simulink model "Sim_Multi"  (R2016b)
settings: Solver=ode3  StartTime=0.0  StopTime=sim_time  FixedStep=t_sim  MaxStep=t_control  RelTol=1e-5  EnableMultiTasking=on
values from neighbouring files (symbols this model uses):
  Att_init = [0;0;0] * d2r    [Init_Multi.m]
  Blade_flapping = 0    [Init_Multi.m]
  C_D = 0.40    (= 0.4)    [Init_Multi.m]
  CoG_nominal = [0;0;0.001]    [Init_Multi.m]
  CoG_real = [0;0;0.001]    [Init_Multi.m]
  Coriolis_correction = 1    [Init_Multi.m]
  d2r = pi/180    (= 0.0174532925199)    [Init_Multi.m]
  Dyn_thrust = 0    [Init_Multi.m]
  g = 9.80665    [Init_Multi.m]
  J_nominal = [Jxx Jxy Jxz;Jyx Jyy Jyz;Jzx Jzy Jzz]    [Init_Multi.m]
  J_real = [Jxx Jxy Jxz;Jyx Jyy Jyz;Jzx Jzy Jzz]    [Init_Multi.m]
  k1 = -1.125    [Init_Multi.m]
  k2 = -1.372    [Init_Multi.m]
  k3 = -1.718    [Init_Multi.m]
  k4 = -0.655    [Init_Multi.m]
  k_a1s = 1.5 / 4.0    (= 0.375)    [Init_Multi.m]
  k_beta = 0.23    [Init_Multi.m]
  kappa = 1.00    (= 1)    [Init_Multi.m]
  Kff_1 = 0.7*[1;1;0.95]    [Init_Multi.m]
  Ki_1 = 10*[1;1;1.5]    [Init_Multi.m]
  Kp_1 = 15*[1;1;1.5]    [Init_Multi.m]
  mass_nominal = 0.550    (= 0.55)    [Init_Multi.m]
  mass_real = 0.550    (= 0.55)    [Init_Multi.m]
  max_thrust = max_thrust + (MotorMatrix_nominal(i,7)*MotorMatrix_nominal(i,12)+MotorMatrix_nominal(i,8)*MotorMatrix_nominal(i,12)^2)    [Init_Multi.m]
  MaxRate_cmd = [360;360;120] * d2r    [Init_Multi.m]
  min_thrust = min_thrust + (MotorMatrix_nominal(i,7)*MotorMatrix_nominal(i,11)+MotorMatrix_nominal(i,8)*MotorMatrix_nominal(i,11)^2)    [Init_Multi.m]
  MotorMap = B' * inv(B * B')    [Init_Multi.m]
  MotorMatrix_nominal = [045 , 0.170 , -0.028 , -1 , 1.0 , 0.010 , [9.6820 , 0.010872]*1e-5 , [1.4504 , 0.0016312]*1e-6 , 0000 , 6000 , [0.0 , 0.0 , 0.0] , 8*2.54/100 , 11/1000;                         135 , 0.170 , -0.028 , +1 , 1.0 , 0.010 , [9.6820 , 0.010872]*1e-5 , [1.4504 , 0.0016312]*1e-6 , 0000 , 6000 , [0.0 , 0.0 , 0.0] , 8*2.54/100 , 11/1000;                         225 , 0.170 , -0.028 , -1 , 1.0 , 0.010 , [9. ...(+284 chars)    [Init_Multi.m]
  MotorMatrix_real = [045 , 0.170 , -0.028 , -1 , 1.0 , 0.010 , [9.6820 , 0.010872]*1e-5 , [1.4504 , 0.0016312]*1e-6 , 0000 , 6000 , [0.0 , 0.0 , 0.0] , 8*2.54/100 , 11/1000;                      135 , 0.170 , -0.028 , +1 , 1.0 , 0.010 , [9.6820 , 0.010872]*1e-5 , [1.4504 , 0.0016312]*1e-6 , 0000 , 6000 , [0.0 , 0.0 , 0.0] , 8*2.54/100 , 11/1000;                      225 , 0.170 , -0.028 , -1 , 1.0 , 0.010 , [9.6820 , ...(+275 chars)    [Init_Multi.m]
  Noise_flag = 0    [Init_Multi.m]
  omega_init = [0;0;0]    [Init_Multi.m]
  q_init = rpy2quat(Att_init)    [Init_Multi.m]
  r2d = 180/pi    (= 57.2957795131)    [Init_Multi.m]
  rho = 1.225    [Init_Multi.m]
  rpm2radpersec = 2*pi/60    (= 0.10471975512)    [Init_Multi.m]
  rpm_init = 3104.5025852    [Init_Multi.m]
  Surface_params = [a;b;c]    [Init_Multi.m]
  t_control = 1/500    (= 0.002)    [Init_Multi.m]
  t_sim = t_control/2    (= 0.001)    [Init_Multi.m]
  thrust_gain = (max_thrust - min_thrust) / 1000    (= 0)    [Init_Multi.m]
  thrust_offset = min_thrust    (= 0)    [Init_Multi.m]
  thrust_reserve = 0.10    (= 0.1)    [Init_Multi.m]
  v_h = 4.0    (= 4)    [Init_Multi.m]
  Vb_init = [0;0;0]    [Init_Multi.m]
  Vi_init = R_IB_init' * Vb_init    [Init_Multi.m]
  Xi_init = [0;0;0]    [Init_Multi.m]
undefined symbols (not defined in the file or in its folder): DiscIntNeverNeededParam, rpy2quat, thrust2rpm
libraries: simulink x17
(part 2 of 4)

== system Sim_Multi/True dynamic system representation of a multirotor UAV/Force//Moment computation/Forces and moments generated by spinning propellers ==
  note: Computation of forces and moments for each actuator specified in the initialization routine
  RPM_commands : Inport
  Dynamic parameters : Inport  Port=2
  6DOF dynamics : Inport  Port=3
  Bus Selector : BusSelector  OutputSignals=omega,V_b,DCM_ib
  Bus Selector1 : BusSelector  OutputSignals=Wind_i,MotorMatrix_real,CoG_real
  For Each Subsystem : Subsystem  TreatAsAtomicUnit=on
  Reshape : Reshape  OutputDimensionality=Column vector (2-D)
  Sum of Elements : Sum  Inputs=+  CollapseMode=Specified dimension  CollapseDim=2
  Sum of Elements1 : Sum  Inputs=+  CollapseMode=Specified dimension  CollapseDim=2
  Total airspeed (Body axes) : Subsystem
  Motor moments : Outport
  Motor forces : Outport  Port=2
  tag scope: RPM_motor=global
  wires:
  For Each Subsystem/1(Motor_force) -> Sum of Elements/1
  For Each Subsystem/2(Motor_moment) -> Sum of Elements1/1
  Sum of Elements/1 -> Motor forces/1
  Sum of Elements1/1 -> Motor moments/1
  RPM_commands/1 -> For Each Subsystem/1(RPM_commands)
  6DOF dynamics/1 -> Bus Selector/1
  Bus Selector/1 -> For Each Subsystem/2(Body_rates)  "<omega>"
  Dynamic parameters/1 -> Bus Selector1/1
  Bus Selector1/2 -> For Each Subsystem/4(MotorMatrix_real)  "<MotorMatrix_real>"
  Bus Selector1/3 -> For Each Subsystem/5(CoG_real)  "<CoG_real>"
  Bus Selector/2 -> Total airspeed (Body axes)/1(V_b)  "<V_b>"
  Bus Selector/3 -> Total airspeed (Body axes)/2(DCM_ib)  "<DCM_ib>"
  Bus Selector1/1 -> Total airspeed (Body axes)/3(Wind_i)  "<Wind_i>"
  Total airspeed (Body axes)/1(Airspeed (Body)) -> For Each Subsystem/3(Airspeed (Body))
  For Each Subsystem/3(RPM_motor) -> Reshape/1
  Reshape/1 -> [RPM_motor]

== system Sim_Multi/Controller/Controller Structure/Inner-loop control only/Conversion stick values to rate commands ==
  Sticks/Throttle cmd : Inport
  Constant : Constant  Value=thrust_offset
  Demux8 : Demux  Outputs=[3 1]
  Mux3 : Mux  Inputs=2
  Sum4 : Sum  Inputs=|++
  Unit conversion [stick value] to [N] : Gain  Gain=thrust_gain
  Unit conversion [stick value] to [rad/s] : Gain  Gain=MaxRate_cmd/500
  Rates/Throttle cmd : Outport
  wires:
  Sticks/Throttle cmd/1 -> Demux8/1
  Demux8/1 -> Unit conversion [stick value] to [rad/s]/1
  Unit conversion [stick value] to [N]/1 -> Sum4/1
  Constant/1 -> Sum4/2
  Demux8/2 -> Unit conversion [stick value] to [N]/1  "Throttle cmd"
  Sum4/1 -> Mux3/2  "Throttle command (thrust value)"
  Mux3/1 -> Rates/Throttle cmd/1
  Unit conversion [stick value] to [rad/s]/1 -> Mux3/1

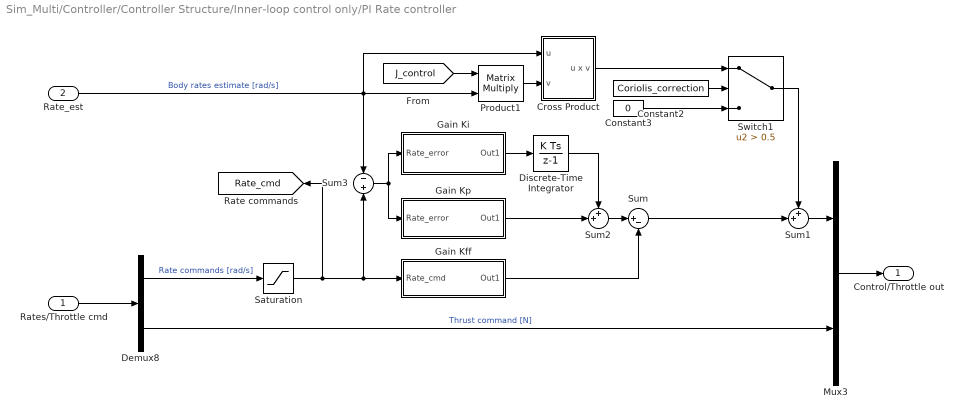
== system Sim_Multi/Controller/Controller Structure/Inner-loop control only/PI Rate controller ==
  Rates/Throttle cmd : Inport
  Rate_est : Inport  Port=2
  Constant2 : Constant  Value=Coriolis_correction
  Constant3 : Constant  Value=0
  Cross Product : Subsystem
  Demux8 : Demux  Outputs=[3 1]
  Discrete-Time Integrator : DiscreteIntegrator  SampleTime=t_control  ICPrevOutput=DiscIntNeverNeededParam  ICPrevScaledInput=DiscIntNeverNeededParam
  Gain Kff : Subsystem
  Gain Ki : Subsystem
  Gain Kp : Subsystem
  Mux3 : Mux  Inputs=2
  Product1 : Product  Multiplication=Matrix(*)  SampleTime=t_control  RndMeth=Zero
  Saturation : Saturate  UpperLimit=MaxRate_cmd  LowerLimit=-MaxRate_cmd
  Sum : Sum  Inputs=|+-
  Sum1 : Sum  Inputs=++|
  Sum2 : Sum  Inputs=++|
  Sum3 : Sum  Inputs=-|+
  Switch1 : Switch  Criteria=u2 > Threshold  Threshold=0.5  SampleTime=t_control
  Control/Throttle out : Outport
  tag scope: Rate_cmd=global
  wires:
  Rate_est/1 -> Product1/2, Sum3/1, Cross Product/1(u)  "Body rates estimate [rad/s]"
  Mux3/1 -> Control/Throttle out/1
  Rates/Throttle cmd/1 -> Demux8/1
  Gain Ki/1(Out1) -> Discrete-Time Integrator/1
  Discrete-Time Integrator/1 -> Sum2/1
  Gain Kp/1(Out1) -> Sum2/2
  [J_control] -> Product1/1
  Product1/1 -> Cross Product/2(v)
  Sum1/1 -> Mux3/1
  Demux8/1 -> Saturation/1  "Rate commands [rad/s]"
  Sum3/1 -> Gain Kp/1(Rate_error), Gain Ki/1(Rate_error)
  Sum/1 -> Sum1/2
  Sum2/1 -> Sum/1
  Gain Kff/1(Out1) -> Sum/2
  Demux8/2 -> Mux3/2  "Thrust command [N]"
  Constant2/1 -> Switch1/2
  Cross Product/1(u x v) -> Switch1/1
  Constant3/1 -> Switch1/3
  Switch1/1 -> Sum1/1
  Saturation/1 -> [Rate_cmd], Sum3/2, Gain Kff/1(Rate_cmd)

== system Sim_Multi/State Estimation, Sensors, Noise/State estimation/Normalize/norm ==
  u : Inport
  Complex to Real-Imag : ComplexToRealImag  Output=Real
  Sqrt : Sqrt  SaturateOnIntegerOverflow=on
  dot_product : Subsystem
  ||u|| : Outport
  wires:
  u/1 -> dot_product/1(u), dot_product/2(v)
  dot_product/1(u.v) -> Sqrt/1
  Sqrt/1 -> Complex to Real-Imag/1
  Complex to Real-Imag/1 -> ||u||/1

== system Sim_Multi/True dynamic system representation of a multirotor UAV/6DOF model/Calculate omega_dot/Cross Product omega x (J * omega) ==
  omega : Inport
  J * omega : Inport  Port=2
  Subsystem : Subsystem
  Subsystem1 : Subsystem
  Sum : Sum  Inputs=+|-
  omega x (J * omega) : Outport
  wires:
  Sum/1 -> omega x (J * omega)/1
  omega/1 -> Subsystem1/1(u), Subsystem/1(u)
  J * omega/1 -> Subsystem/2(v), Subsystem1/2(v)
  Subsystem/1(Positive elements) -> Sum/1
  Subsystem1/1(Negative elements) -> Sum/2

== system Sim_Multi/True dynamic system representation of a multirotor UAV/6DOF model/Calculate omega_dot/Subsystem ==
  omega : Inport
  J : Inport  Port=2
  Product : Product  Multiplication=Matrix(*)
  Reshape : Reshape  OutputDimensionality=Column vector (2-D)
  Reshape1 : Reshape  OutputDimensionality=Column vector (2-D)
  J * omega : Outport
  wires:
  Reshape1/1 -> J * omega/1
  Product/1 -> Reshape1/1
  J/1 -> Product/1
  Reshape/1 -> Product/2
  omega/1 -> Reshape/1

== system Sim_Multi/True dynamic system representation of a multirotor UAV/6DOF model/Quat Strapdown Eq./Cross Product ==
  u : Inport
  v : Inport  Port=2
  Subsystem : Subsystem
  Subsystem1 : Subsystem
  Sum : Sum  Inputs=+|-
  u x v : Outport
  wires:
  Sum/1 -> u x v/1
  u/1 -> Subsystem1/1(u), Subsystem/1(u)
  v/1 -> Subsystem1/2(v), Subsystem/2(v)
  Subsystem/1(Positive elements) -> Sum/1
  Subsystem1/1(Negative elements) -> Sum/2

== system Sim_Multi/True dynamic system representation of a multirotor UAV/6DOF model/Quat Strapdown Eq./Dot product ==
  u : Inport
  v : Inport  Port=2
  Product : Product  Multiplication=Matrix(*)  RndMeth=Zero
  Reshape : Reshape  OutputDimensionality=Column vector (2-D)
  Reshape1 : Reshape  OutputDimensionality=Column vector (2-D)
  transpose : Math  Operator=transpose  SaturateOnIntegerOverflow=on
  u.v : Outport
  wires:
  v/1 -> Reshape1/1
  u/1 -> Reshape/1
  Reshape/1 -> transpose/1
  transpose/1 -> Product/1
  Reshape1/1 -> Product/2
  Product/1 -> u.v/1

== system Sim_Multi/True dynamic system representation of a multirotor UAV/6DOF model/Quat Strapdown Eq./Normalize ==
  Input : Inport
  Divide : Product  Inputs=*/
  norm : Subsystem
  Output : Outport
  wires:
  Input/1 -> Divide/1, norm/1(u)
  norm/1(||u||) -> Divide/2
  Divide/1 -> Output/1

== system Sim_Multi/True dynamic system representation of a multirotor UAV/6DOF model/Quat to Rotation Matrix/Subsystem ==
  q : Inport
  Add : Sum  Inputs=++--
  Demux : Demux
  Product{,2..4} (4 alike) : Product
  C_11 : Outport
  wires:
  Product2/1 -> Add/2
  Product4/1 -> Add/4
  Add/1 -> C_11/1
  Demux/2 -> Product2/2, Product2/1
  Product3/1 -> Add/3
  Demux/3 -> Product3/2, Product3/1
  Demux/1 -> Product/2, Product/1
  q/1 -> Demux/1
  Product/1 -> Add/1
  Demux/4 -> Product4/2, Product4/1

== system Sim_Multi/True dynamic system representation of a multirotor UAV/6DOF model/Quat to Rotation Matrix/Subsystem1 ==
  q : Inport
  Add : Sum  Inputs=+-+-
  Demux : Demux
  Product{,2..4} (4 alike) : Product
  C_22 : Outport
  wires:
  Product2/1 -> Add/2
  Product4/1 -> Add/4
  Add/1 -> C_22/1
  Demux/2 -> Product2/2, Product2/1
  Product3/1 -> Add/3
  Demux/3 -> Product3/2, Product3/1
  Demux/1 -> Product/2, Product/1
  q/1 -> Demux/1
  Product/1 -> Add/1
  Demux/4 -> Product4/2, Product4/1

== system Sim_Multi/True dynamic system representation of a multirotor UAV/6DOF model/Quat to Rotation Matrix/Subsystem2 ==
  q : Inport
  Add : Sum  Inputs=+--+
  Demux : Demux
  Product{,2..4} (4 alike) : Product
  C_33 : Outport
  wires:
  Product2/1 -> Add/2
  Product4/1 -> Add/4
  Add/1 -> C_33/1
  Demux/2 -> Product2/2, Product2/1
  Product3/1 -> Add/3
  Demux/3 -> Product3/2, Product3/1
  Demux/1 -> Product/2, Product/1
  q/1 -> Demux/1
  Product/1 -> Add/1
  Demux/4 -> Product4/2, Product4/1

== system Sim_Multi/True dynamic system representation of a multirotor UAV/6DOF model/Quat to Rotation Matrix/Subsystem3 ==
  q : Inport
  Add : Sum
  Demux : Demux
  Gain : Gain  Gain=2
  Product : Product
  Product2 : Product
  C_12 : Outport
  wires:
  Add/1 -> Gain/1
  q/1 -> Demux/1
  Demux/2 -> Product/1
  Demux/3 -> Product/2
  Demux/1 -> Product2/1
  Demux/4 -> Product2/2
  Product/1 -> Add/1
  Product2/1 -> Add/2
  Gain/1 -> C_12/1

== system Sim_Multi/True dynamic system representation of a multirotor UAV/6DOF model/Quat to Rotation Matrix/Subsystem4 ==
  q : Inport
  Add : Sum  Inputs=+-
  Demux : Demux
  Gain : Gain  Gain=2
  Product : Product
  Product2 : Product
  C_13 : Outport
  wires:
  Add/1 -> Gain/1
  q/1 -> Demux/1
  Product/1 -> Add/1
  Product2/1 -> Add/2
  Gain/1 -> C_13/1
  Demux/2 -> Product/1
  Demux/4 -> Product/2
  Demux/1 -> Product2/1
  Demux/3 -> Product2/2

== system Sim_Multi/True dynamic system representation of a multirotor UAV/6DOF model/Quat to Rotation Matrix/Subsystem5 ==
  q : Inport
  Add : Sum  Inputs=+-
  Demux : Demux
  Gain : Gain  Gain=2
  Product : Product
  Product2 : Product
  C_21 : Outport
  wires:
  Add/1 -> Gain/1
  q/1 -> Demux/1
  Product/1 -> Add/1
  Product2/1 -> Add/2
  Gain/1 -> C_21/1
  Demux/2 -> Product/1
  Demux/3 -> Product/2
  Demux/1 -> Product2/1
  Demux/4 -> Product2/2

== system Sim_Multi/True dynamic system representation of a multirotor UAV/6DOF model/Quat to Rotation Matrix/Subsystem6 ==
  q : Inport
  Add : Sum
  Demux : Demux
  Gain : Gain  Gain=2
  Product : Product
  Product2 : Product
  C_23 : Outport
  wires:
  Add/1 -> Gain/1
  q/1 -> Demux/1
  Product/1 -> Add/1
  Product2/1 -> Add/2
  Gain/1 -> C_23/1
  Demux/3 -> Product/1
  Demux/4 -> Product/2
  Demux/1 -> Product2/1
  Demux/2 -> Product2/2

== system Sim_Multi/True dynamic system representation of a multirotor UAV/6DOF model/Quat to Rotation Matrix/Subsystem7 ==
  q : Inport
  Add : Sum
  Demux : Demux
  Gain : Gain  Gain=2
  Product : Product
  Product2 : Product
  C_31 : Outport
  wires:
  Add/1 -> Gain/1
  q/1 -> Demux/1
  Product/1 -> Add/1
  Product2/1 -> Add/2
  Gain/1 -> C_31/1
  Demux/2 -> Product/1
  Demux/4 -> Product/2
  Demux/1 -> Product2/1
  Demux/3 -> Product2/2

== system Sim_Multi/True dynamic system representation of a multirotor UAV/6DOF model/Quat to Rotation Matrix/Subsystem8 ==
  q : Inport
  Add : Sum  Inputs=+-
  Demux : Demux
  Gain : Gain  Gain=2
  Product : Product
  Product2 : Product
  C_32 : Outport
  wires:
  Add/1 -> Gain/1
  q/1 -> Demux/1
  Product/1 -> Add/1
  Product2/1 -> Add/2
  Gain/1 -> C_32/1
  Demux/3 -> Product/1
  Demux/4 -> Product/2
  Demux/1 -> Product2/1
  Demux/2 -> Product2/2

== system Sim_Multi/True dynamic system representation of a multirotor UAV/6DOF model/Quat to Rotation Matrix/Subsystem9 ==
  C_11 : Inport  PortDimensions=1
  C_12 : Inport  Port=2  PortDimensions=1
  C_13 : Inport  Port=3  PortDimensions=1
  C_21 : Inport  Port=4  PortDimensions=1
  C_22 : Inport  Port=5  PortDimensions=1
  C_23 : Inport  Port=6  PortDimensions=1
  C_31 : Inport  Port=7  PortDimensions=1
  C_32 : Inport  Port=8  PortDimensions=1
  C_33 : Inport  Port=9  PortDimensions=1
  Reshape (9) to [3x3] column-major : Reshape  OutputDimensionality=Customize  OutputDimensions=[3,3]
  Vector Concatenate : Concatenate  NumInputs=9
  DCM_ib : Outport
  wires:
  C_33/1 -> Vector Concatenate/9
  C_22/1 -> Vector Concatenate/5
  Reshape (9) to [3x3] column-major/1 -> DCM_ib/1
  C_11/1 -> Vector Concatenate/1
  Vector Concatenate/1 -> Reshape (9) to [3x3] column-major/1
  C_32/1 -> Vector Concatenate/6
  C_31/1 -> Vector Concatenate/3
  C_21/1 -> Vector Concatenate/2
  C_13/1 -> Vector Concatenate/7
  C_12/1 -> Vector Concatenate/4
  C_23/1 -> Vector Concatenate/8

== system Sim_Multi/True dynamic system representation of a multirotor UAV/6DOF model/omega x V_b/Subsystem ==
  u : Inport
  v : Inport  Port=2
  Demux : Demux  Outputs=3
  Demux1 : Demux  Outputs=3
  Mux : Mux  Inputs=3
  Product : Product
  Product1 : Product
  Product2 : Product
  Positive elements : Outport
  wires:
  Mux/1 -> Positive elements/1
  v/1 -> Demux1/1
  u/1 -> Demux/1
  Demux/2 -> Product/1
  Demux1/3 -> Product/2
  Demux/3 -> Product1/1
  Demux1/1 -> Product1/2
  Demux/1 -> Product2/1
  Demux1/2 -> Product2/2
  Product/1 -> Mux/1  "u2*v3"
  Product1/1 -> Mux/2  "u3*v1"
  Product2/1 -> Mux/3  "u1*v2"

== system Sim_Multi/True dynamic system representation of a multirotor UAV/6DOF model/omega x V_b/Subsystem1 ==
  u : Inport
  v : Inport  Port=2
  Demux : Demux  Outputs=3
  Demux1 : Demux  Outputs=3
  Mux : Mux  Inputs=3
  Product : Product
  Product1 : Product
  Product2 : Product
  Negative elements : Outport
  wires:
  Mux/1 -> Negative elements/1
  v/1 -> Demux1/1
  u/1 -> Demux/1
  Product/1 -> Mux/1  "u3*v2"
  Product1/1 -> Mux/2  "u1*v3"
  Product2/1 -> Mux/3  "u2*v1"
  Demux/3 -> Product/1
  Demux1/2 -> Product/2
  Demux/1 -> Product1/1
  Demux1/3 -> Product1/2
  Demux/2 -> Product2/1
  Demux1/1 -> Product2/2

== system Sim_Multi/True dynamic system representation of a multirotor UAV/Force//Moment computation/Compute aerodynamic drag of the airframe in Body axes/Aerodynamic drag force ==
  note: This block computes the surface area of the airframe that is visible in the direction of the airspeed.
      | Drag force is computed by the standard drag equation: 1/2*rho*u^2*C_D*A
  Airspeed (Body axes) : Inport
  Surface_params : Inport  Port=2
  If : If  IfExpression=u1 == 0
  Merge : Merge
  Nonzero airspeed : Subsystem  TreatAsAtomicUnit=on
  Zero airspeed : Subsystem  TreatAsAtomicUnit=on
  norm : Subsystem
  Drag force (Body axes) : Outport
  wires:
  If/1 -> Zero airspeed/Action
  Zero airspeed/1(Drag force) -> Merge/1
  Nonzero airspeed/1(Drag force) -> Merge/2
  If/2 -> Nonzero airspeed/Action
  Airspeed (Body axes)/1 -> norm/1(u), Nonzero airspeed/1(Airspeed (Body)), Zero airspeed/1(Airspeed)
  norm/1(||u||) -> If/1  "Airspeed magnitude"
  Merge/1 -> Drag force (Body axes)/1  "Force against direction of motion due to aerodynamic drag"
  Surface_params/1 -> Nonzero airspeed/2(Surface_params), Zero airspeed/2(Surface_params)

== system Sim_Multi/True dynamic system representation of a multirotor UAV/Force//Moment computation/Compute aerodynamic drag of the airframe in Body axes/Total airspeed (Body axes) ==
  V_b : Inport
  DCM_ib : Inport  Port=2
  Wind_i : Inport  Port=3
  Inertial to Body : Subsystem
  Reshape : Reshape  OutputDimensionality=Column vector (2-D)
  Sum1 : Sum  Inputs=|+-
  Airspeed (Body) : Outport
  wires:
  DCM_ib/1 -> Inertial to Body/1(DCM_ib)
  Wind_i/1 -> Inertial to Body/2(Wind_i)
  Inertial to Body/1(Wind_b) -> Sum1/2  "Wind velocity (Body axes)"
  Reshape/1 -> Sum1/1
  V_b/1 -> Reshape/1
  Sum1/1 -> Airspeed (Body)/1  "True airspeed (Body axes)"

== system Sim_Multi/True dynamic system representation of a multirotor UAV/Force//Moment computation/Forces and moments generated by spinning propellers/For Each Subsystem ==
  note: This subsystem computes all the forces and moments generated by each of the actuators.
      |
      | That includes dynamic thrust, blade flapping effects, gyroscopic moments, and others.
      | All forces and moments are computed as acting on the real center of gravity of the airframe,
      | which might change during the simulation due to failure cases or the dropping of cargo.
      |
      | Outputs are the total force and moment vectors for each one of the motors.
  RPM_commands : Inport  Partition=on  PartitionDimension=1  PartitionWidth=1
  Body_rates : Inport  Port=2
  Airspeed (Body) : Inport  Port=3
  MotorMatrix_real : Inport  Port=4  Partition=on  PartitionDimension=1  PartitionWidth=1
  CoG_real : Inport  Port=5
  Actuator dynamics : Subsystem
  Cross Product : Subsystem
  For Each : ForEach  DisableCoverage=on  IndexMode=One-based
  Leverarm vector from real CoG to each propeller (Body axes) : Subsystem
  Rate Transition : RateTransition  OutPortSampleTime=t_sim
  Sum1 : Sum  Inputs=|++
  Thrust/moment vector for each propeller (Body axes) : Subsystem
  Motor_force : Outport  ConcatenationDimension=2
  Motor_moment : Outport  Port=2  ConcatenationDimension=2
  RPM_motor : Outport  Port=3  ConcatenationDimension=2
  wires:
  Leverarm vector from real CoG to each propeller (Body axes)/1(Prop_vector) -> Cross Product/1(r), Thrust/moment vector for each propeller (Body axes)/1(Prop_vector)  "Leverarm vector from real CoG to propeller (Body axes)"
  MotorMatrix_real/1 -> Leverarm vector from real CoG to each propeller (Body axes)/1(MotorMatrix_real), Thrust/moment vector for each propeller (Body axes)/4(MotorMatrix_real), Actuator dynamics/1(MotorMatrix_real)
  Thrust/moment vector for each propeller (Body axes)/1(Thrust_vector (Body axes)) -> Motor_force/1  "Thrust force vector for each motor (Body axes)"
  Thrust/moment vector for each propeller (Body axes)/2(Motor_moments (Body axes)) -> Motor_moment/1  "Moment vector for each motor (Body axes)"
  RPM_commands/1 -> Rate Transition/1
  Body_rates/1 -> Thrust/moment vector for each propeller (Body axes)/3(Body_rates), Cross Product/2(omega)
  CoG_real/1 -> Leverarm vector from real CoG to each propeller (Body axes)/2(CoG_real)
  Cross Product/1(omega x r) -> Sum1/1  "Linear velocity at prop due to body angular rates (Body axes)"
  Airspeed (Body)/1 -> Sum1/2  "True linear velocity of airframe (including wind) (Body axes)"
  Sum1/1 -> Thrust/moment vector for each propeller (Body axes)/2(True airspeed)  "Total linear velocity at prop (Body axes)"
  Actuator dynamics/1(RPM_motor) -> RPM_motor/1, Thrust/moment vector for each propeller (Body axes)/5(RPM_motor)  "Actual motor RPM"
  Rate Transition/1 -> Actuator dynamics/2(RPM_command)

== system Sim_Multi/True dynamic system representation of a multirotor UAV/Force//Moment computation/Forces and moments generated by spinning propellers/Total airspeed (Body axes) ==
  V_b : Inport
  DCM_ib : Inport  Port=2
  Wind_i : Inport  Port=3
  Inertial to Body : Subsystem
  Reshape : Reshape  OutputDimensionality=Column vector (2-D)
  Sum1 : Sum  Inputs=|+-
  Airspeed (Body) : Outport
  wires:
  DCM_ib/1 -> Inertial to Body/1(DCM_ib)
  Wind_i/1 -> Inertial to Body/2(Wind_i)
  Inertial to Body/1(Wind_b) -> Sum1/2  "Wind velocity (Body axes)"
  Sum1/1 -> Airspeed (Body)/1  "True airspeed (Body axes)"
  Reshape/1 -> Sum1/1
  V_b/1 -> Reshape/1

== system Sim_Multi/Controller/Controller Structure/Inner-loop control only/PI Rate controller/Cross Product ==
  u : Inport
  v : Inport  Port=2
  Subsystem : Subsystem
  Subsystem1 : Subsystem
  Sum : Sum  Inputs=+|-
  u x v : Outport
  wires:
  Sum/1 -> u x v/1
  u/1 -> Subsystem1/1(u), Subsystem/1(u)
  v/1 -> Subsystem1/2(v), Subsystem/2(v)
  Subsystem/1(Positive elements) -> Sum/1
  Subsystem1/1(Negative elements) -> Sum/2

== system Sim_Multi/Controller/Controller Structure/Inner-loop control only/PI Rate controller/Gain Kff ==
  Rate_cmd : Inport
  Constant1 : Constant  Value=Kff_1
  Create diagonal 3x3 matrix : Subsystem
  Product : Product  Multiplication=Matrix(*)  SampleTime=t_control  RndMeth=Zero
  Product1 : Product  Multiplication=Matrix(*)  RndMeth=Zero
  Out1 : Outport
  wires:
  [J_control] -> Product1/1
  Product1/1 -> Product/1
  Rate_cmd/1 -> Product/2
  Constant1/1 -> Create diagonal 3x3 matrix/1(Vector)
  Create diagonal 3x3 matrix/1(Matrix) -> Product1/2
  Product/1 -> Out1/1

== system Sim_Multi/Controller/Controller Structure/Inner-loop control only/PI Rate controller/Gain Ki ==
  Rate_error : Inport
  Constant1 : Constant  Value=Ki_1
  Create diagonal 3x3 matrix : Subsystem
  Product : Product  Multiplication=Matrix(*)  SampleTime=t_control  RndMeth=Zero
  Product1 : Product  Multiplication=Matrix(*)  RndMeth=Zero
  Out1 : Outport
  wires:
  [J_control] -> Product1/1
  Product1/1 -> Product/1
  Rate_error/1 -> Product/2
  Constant1/1 -> Create diagonal 3x3 matrix/1(Vector)
  Create diagonal 3x3 matrix/1(Matrix) -> Product1/2
  Product/1 -> Out1/1

== system Sim_Multi/Controller/Controller Structure/Inner-loop control only/PI Rate controller/Gain Kp ==
  Rate_error : Inport
  Constant1 : Constant  Value=Kp_1
  Create diagonal 3x3 matrix : Subsystem
  Product : Product  Multiplication=Matrix(*)  SampleTime=t_control  RndMeth=Zero
  Product1 : Product  Multiplication=Matrix(*)  RndMeth=Zero
  Out1 : Outport
  wires:
  [J_control] -> Product1/1
  Product1/1 -> Product/1
  Rate_error/1 -> Product/2
  Constant1/1 -> Create diagonal 3x3 matrix/1(Vector)
  Create diagonal 3x3 matrix/1(Matrix) -> Product1/2
  Product/1 -> Out1/1

== system Sim_Multi/State Estimation, Sensors, Noise/State estimation/Normalize/norm/dot_product ==
  u : Inport
  v : Inport  Port=2
  Product : Product  Multiplication=Matrix(*)  RndMeth=Zero
  Reshape : Reshape  OutputDimensionality=Column vector (2-D)
  Reshape1 : Reshape  OutputDimensionality=Column vector (2-D)
  transpose : Math  Operator=transpose  SaturateOnIntegerOverflow=on
  u.v : Outport
  wires:
  v/1 -> Reshape1/1
  u/1 -> Reshape/1
  Reshape/1 -> transpose/1
  transpose/1 -> Product/1
  Reshape1/1 -> Product/2
  Product/1 -> u.v/1

== system Sim_Multi/True dynamic system representation of a multirotor UAV/6DOF model/Calculate omega_dot/Cross Product omega x (J * omega)/Subsystem ==
  u : Inport
  v : Inport  Port=2
  Demux : Demux  Outputs=3
  Demux1 : Demux  Outputs=3
  Mux : Mux  Inputs=3
  Product : Product
  Product1 : Product
  Product2 : Product
  Positive elements : Outport
  wires:
  Mux/1 -> Positive elements/1
  v/1 -> Demux1/1
  u/1 -> Demux/1
  Demux/2 -> Product/1
  Demux1/3 -> Product/2
  Demux/3 -> Product1/1
  Demux1/1 -> Product1/2
  Demux/1 -> Product2/1
  Demux1/2 -> Product2/2
  Product/1 -> Mux/1  "u2*v3"
  Product1/1 -> Mux/2  "u3*v1"
  Product2/1 -> Mux/3  "u1*v2"

== system Sim_Multi/True dynamic system representation of a multirotor UAV/6DOF model/Calculate omega_dot/Cross Product omega x (J * omega)/Subsystem1 ==
  u : Inport
  v : Inport  Port=2
  Demux : Demux  Outputs=3
  Demux1 : Demux  Outputs=3
  Mux : Mux  Inputs=3
  Product : Product
  Product1 : Product
  Product2 : Product
  Negative elements : Outport
  wires:
  Mux/1 -> Negative elements/1
  v/1 -> Demux1/1
  u/1 -> Demux/1
  Product/1 -> Mux/1  "u3*v2"
  Product1/1 -> Mux/2  "u1*v3"
  Product2/1 -> Mux/3  "u2*v1"
  Demux/3 -> Product/1
  Demux1/2 -> Product/2
  Demux/1 -> Product1/1
  Demux1/3 -> Product1/2
  Demux/2 -> Product2/1
  Demux1/1 -> Product2/2

== system Sim_Multi/True dynamic system representation of a multirotor UAV/6DOF model/Quat Strapdown Eq./Cross Product/Subsystem ==
  u : Inport
  v : Inport  Port=2
  Demux : Demux  Outputs=3
  Demux1 : Demux  Outputs=3
  Mux : Mux  Inputs=3
  Product : Product
  Product1 : Product
  Product2 : Product
  Positive elements : Outport
  wires:
  Mux/1 -> Positive elements/1
  v/1 -> Demux1/1
  u/1 -> Demux/1
  Demux/2 -> Product/1
  Demux1/3 -> Product/2
  Demux/3 -> Product1/1
  Demux1/1 -> Product1/2
  Demux/1 -> Product2/1
  Demux1/2 -> Product2/2
  Product/1 -> Mux/1  "u2*v3"
  Product1/1 -> Mux/2  "u3*v1"
  Product2/1 -> Mux/3  "u1*v2"

== system Sim_Multi/True dynamic system representation of a multirotor UAV/6DOF model/Quat Strapdown Eq./Cross Product/Subsystem1 ==
  u : Inport
  v : Inport  Port=2
  Demux : Demux  Outputs=3
  Demux1 : Demux  Outputs=3
  Mux : Mux  Inputs=3
  Product : Product
  Product1 : Product
  Product2 : Product
  Negative elements : Outport
  wires:
  Mux/1 -> Negative elements/1
  v/1 -> Demux1/1
  u/1 -> Demux/1
  Product/1 -> Mux/1  "u3*v2"
  Product1/1 -> Mux/2  "u1*v3"
  Product2/1 -> Mux/3  "u2*v1"
  Demux/3 -> Product/1
  Demux1/2 -> Product/2
  Demux/1 -> Product1/1
  Demux1/3 -> Product1/2
  Demux/2 -> Product2/1
  Demux1/1 -> Product2/2

== system Sim_Multi/True dynamic system representation of a multirotor UAV/6DOF model/Quat Strapdown Eq./Normalize/norm ==
  u : Inport
  Complex to Real-Imag : ComplexToRealImag  Output=Real
  Sqrt : Sqrt  SaturateOnIntegerOverflow=on
  dot_product : Subsystem
  ||u|| : Outport
  wires:
  u/1 -> dot_product/1(u), dot_product/2(v)
  dot_product/1(u.v) -> Sqrt/1
  Sqrt/1 -> Complex to Real-Imag/1
  Complex to Real-Imag/1 -> ||u||/1

== system Sim_Multi/True dynamic system representation of a multirotor UAV/Force//Moment computation/Compute aerodynamic drag of the airframe in Body axes/Aerodynamic drag force/Nonzero airspeed ==
  Airspeed (Body) : Inport
  Surface_params : Inport  Port=2
  Action Port : ActionPort  ActionType=else
  Abs : Abs
  Constant : Constant  Value=1/2
  Constant1 : Constant  Value=rho
  Constant2 : Constant  Value=C_D
  Drag force opposes direction of airspeed : Gain  Gain=-1
  Normalize : Subsystem
  Product : Product  Inputs=5
  Product1 : Product
  Surface area computation : Subsystem
  u^2 : Subsystem
  Drag force : Outport
  wires:
  Airspeed (Body)/1 -> Surface area computation/1(Airspeed (Body)), Normalize/1(Input), u^2/1(u)
  Surface_params/1 -> Surface area computation/2(Surface_params)
  Constant/1 -> Product/1
  Constant1/1 -> Product/2
  u^2/1(u^2) -> Product/3
  Constant2/1 -> Product/4
  Surface area computation/1(Area) -> Product/5
  Normalize/1(Output) -> Product1/1  "Normalized airspeed vector (Body axes)"
  Product1/1 -> Drag force opposes direction of airspeed/1
  Drag force opposes direction of airspeed/1 -> Drag force/1
  Product/1 -> Abs/1
  Abs/1 -> Product1/2  "Magnitude of drag force"

== system Sim_Multi/True dynamic system representation of a multirotor UAV/Force//Moment computation/Compute aerodynamic drag of the airframe in Body axes/Aerodynamic drag force/Zero airspeed ==
  Airspeed : Inport
  Surface_params : Inport  Port=2
  Action Port : ActionPort  ActionType=then
  Constant : Constant  Value=[0;0;0]
  Terminator : Terminator
  Terminator1 : Terminator
  Drag force : Outport  InitialOutput=[0;0;-1]
  wires:
  Airspeed/1 -> Terminator/1  "Airspeed components in (unbent) rotor plane"
  Constant/1 -> Drag force/1
  Surface_params/1 -> Terminator1/1

== system Sim_Multi/True dynamic system representation of a multirotor UAV/Force//Moment computation/Compute aerodynamic drag of the airframe in Body axes/Aerodynamic drag force/norm ==
  u : Inport
  Complex to Real-Imag : ComplexToRealImag  Output=Real
  Sqrt : Sqrt  SaturateOnIntegerOverflow=on
  dot_product : Subsystem
  ||u|| : Outport
  wires:
  u/1 -> dot_product/1(u), dot_product/2(v)
  dot_product/1(u.v) -> Sqrt/1
  Sqrt/1 -> Complex to Real-Imag/1
  Complex to Real-Imag/1 -> ||u||/1

== system Sim_Multi/True dynamic system representation of a multirotor UAV/Force//Moment computation/Compute aerodynamic drag of the airframe in Body axes/Total airspeed (Body axes)/Inertial to Body ==
  DCM_ib : Inport
  Wind_i : Inport  Port=2
  Product : Product  Multiplication=Matrix(*)
  Reshape : Reshape  OutputDimensionality=Column vector (2-D)
  Reshape1 : Reshape  OutputDimensionality=Column vector (2-D)
  Wind_b : Outport
  wires:
  Reshape/1 -> Product/2
  Product/1 -> Reshape1/1
  Reshape1/1 -> Wind_b/1
  Wind_i/1 -> Reshape/1
  DCM_ib/1 -> Product/1  "DCM_ib"

== system Sim_Multi/True dynamic system representation of a multirotor UAV/Force//Moment computation/Forces and moments generated by spinning propellers/For Each Subsystem/Actuator dynamics ==
  note: This block diagram expresses the actuator dynamics of a specific motor/propeller combination
      | as a first order transfer function. The time constant and gain of this first order transfer function
      | for each motor is listed in the motor matrix.
      | In addition, upper and lower limits of the motor RPM can be set so that the motor output
      | never exceeds those values.
  MotorMatrix_real : Inport
  RPM_command : Inport  Port=2
  Continuous Integrator with dynamic upper/lower limits : Subsystem
  Divide : Product  Inputs=*/
  Product : Product  SampleTime=t_sim  RndMeth=Zero
  Selector : Selector  InputPortWidth=17  IndexOptions=Index vector (dialog)  Indices=[5]  OutputSizes=1
  Selector1 : Selector  InputPortWidth=17  IndexOptions=Index vector (dialog)  Indices=[6]  OutputSizes=1
  Selector2 : Selector  InputPortWidth=17  IndexOptions=Index vector (dialog)  Indices=[11]  OutputSizes=1
  Selector3 : Selector  InputPortWidth=17  IndexOptions=Index vector (dialog)  Indices=[12]  OutputSizes=1
  Sum1 : Sum  Inputs=-+|
  RPM_motor : Outport
  wires:
  Sum1/1 -> Divide/1
  Selector1/1 -> Divide/2  "TF time constant"
  Product/1 -> Sum1/2
  Selector/1 -> Product/2  "TF gain"
  RPM_command/1 -> Product/1
  MotorMatrix_real/1 -> Selector3/1, Selector2/1, Selector1/1, Selector/1
  Divide/1 -> Continuous Integrator with dynamic upper/lower limits/1(Integrator input)
  Continuous Integrator with dynamic upper/lower limits/1(Output) -> RPM_motor/1, Sum1/1
  Selector2/1 -> Continuous Integrator with dynamic upper/lower limits/2(Lower limit)  "RPM min value"
  Selector3/1 -> Continuous Integrator with dynamic upper/lower limits/3(Upper limit)  "RPM max value"

== system Sim_Multi/True dynamic system representation of a multirotor UAV/Force//Moment computation/Forces and moments generated by spinning propellers/For Each Subsystem/Cross Product ==
  r : Inport
  omega : Inport  Port=2
  Reshape : Reshape  OutputDimensionality=Column vector (2-D)
  Subsystem : Subsystem
  Subsystem1 : Subsystem
  Sum : Sum  Inputs=+|-
  omega x r : Outport
  wires:
  Sum/1 -> Reshape/1
  omega/1 -> Subsystem1/1(omega), Subsystem/1(omega)
  r/1 -> Subsystem1/2(r), Subsystem/2(r)
  Subsystem/1(Positive elements) -> Sum/1
  Subsystem1/1(Negative elements) -> Sum/2
  Reshape/1 -> omega x r/1

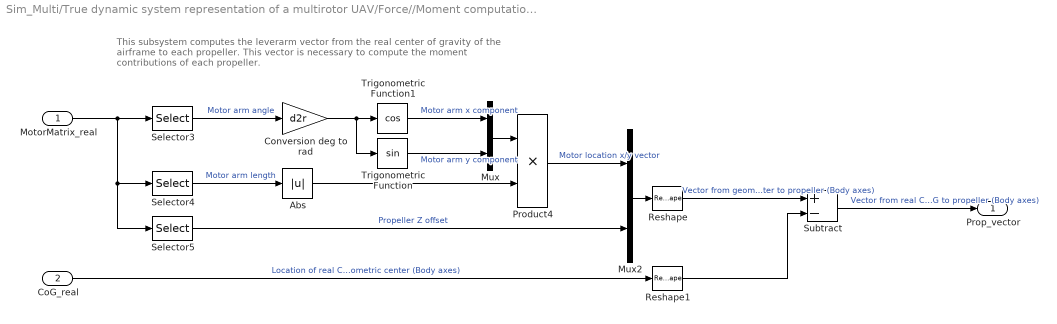
== system Sim_Multi/True dynamic system representation of a multirotor UAV/Force//Moment computation/Forces and moments generated by spinning propellers/For Each Subsystem/Leverarm vector from real CoG to each propeller (Body axes) ==
  note: This subsystem computes the leverarm vector from the real center of gravity
      | of the airframe to each propeller.
      | This vector is necessary to compute the moment contributions of each propeller.
  MotorMatrix_real : Inport
  CoG_real : Inport  Port=2
  Abs : Abs
  Conversion deg to rad : Gain  Gain=d2r
  Mux : Mux  Inputs=2
  Mux2 : Mux  Inputs=2
  Product4 : Product
  Reshape : Reshape  OutputDimensionality=Column vector (2-D)
  Reshape1 : Reshape  OutputDimensionality=Column vector (2-D)
  Selector3 : Selector  InputPortWidth=17  IndexOptions=Index vector (dialog)  Indices=[1]  OutputSizes=1
  Selector4 : Selector  InputPortWidth=17  IndexOptions=Index vector (dialog)  Indices=[2]  OutputSizes=1
  Selector5 : Selector  InputPortWidth=17  IndexOptions=Index vector (dialog)  Indices=[3]  OutputSizes=1
  Subtract : Sum  Inputs=+-
  Trigonometric Function : Trigonometry
  Trigonometric Function1 : Trigonometry  Operator=cos
  Prop_vector : Outport
  wires:
  Selector3/1 -> Conversion deg to rad/1  "Motor arm angle"
  Selector4/1 -> Abs/1  "Motor arm length"
  Selector5/1 -> Mux2/2  "Propeller Z offset"
  Conversion deg to rad/1 -> Trigonometric Function/1, Trigonometric Function1/1
  Trigonometric Function1/1 -> Mux/1  "Motor arm x component"
  Trigonometric Function/1 -> Mux/2  "Motor arm y component"
  Mux/1 -> Product4/1
  Abs/1 -> Product4/2
  Product4/1 -> Mux2/1  "Motor location x/y vector"
  Mux2/1 -> Reshape/1
  CoG_real/1 -> Reshape1/1  "Location of real CoG w.r.t. geometric center (Body axes)"
  Reshape/1 -> Subtract/1  "Vector from geometric center to propeller (Body axes)"
  Reshape1/1 -> Subtract/2
  Subtract/1 -> Prop_vector/1  "Vector from real CoG to propeller (Body axes)"
  MotorMatrix_real/1 -> Selector5/1, Selector4/1, Selector3/1

== system Sim_Multi/True dynamic system representation of a multirotor UAV/Force//Moment computation/Forces and moments generated by spinning propellers/For Each Subsystem/Thrust//moment vector for each propeller (Body axes) ==
  Prop_vector : Inport
  True airspeed : Inport  Port=2
  Body_rates : Inport  Port=3
  MotorMatrix_real : Inport  Port=4
  RPM_motor : Inport  Port=5
  Add : Sum  Inputs=++++
  Compute dynamic motor thrust and moments : Subsystem
  Coordinate transformation Body to Motor axes : Subsystem
  Cross Product : Subsystem
  Reshape : Reshape  OutputDimensionality=Column vector (2-D)
  Thrust_vector (Body axes) : Outport
  Motor_moments (Body axes) : Outport  Port=2
  wires:
  MotorMatrix_real/1 -> Coordinate transformation Body to Motor axes/1(MotorMatrix_real), Compute dynamic motor thrust and moments/2(MotorMatrix_real)
  True airspeed/1 -> Coordinate transformation Body to Motor axes/2(Airspeed (Body axes))
  Coordinate transformation Body to Motor axes/2(Airspeed (Motor axes)) -> Compute dynamic motor thrust and moments/4(Airspeed (Motor axes))
  RPM_motor/1 -> Compute dynamic motor thrust and moments/1(RPM_motor)
  Body_rates/1 -> Compute dynamic motor thrust and moments/5(Body_rates)
  Compute dynamic motor thrust and moments/3(Gyro moment (Body axes)) -> Add/3  "Gyroscopic moments per motor (Body axes)"
  Compute dynamic motor thrust and moments/1(Induced motor moment (Body axes)) -> Add/1  "Induced motor moment at dynamic conditions (Body axes)"
  Add/1 -> Motor_moments (Body axes)/1
  Coordinate transformation Body to Motor axes/1(R_mb) -> Compute dynamic motor thrust and moments/3(R_mb)
  Compute dynamic motor thrust and moments/4(Thrust_vector (Body axes)) -> Thrust_vector (Body axes)/1, Cross Product/2(v)
  Compute dynamic motor thrust and moments/2(Motor hub moment (Body axes)) -> Add/2  "Moment induced in motor hub due to blade flapping (Body axes)"
  Cross Product/1(u x v) -> Reshape/1
  Prop_vector/1 -> Cross Product/1(u)
  Reshape/1 -> Add/4

== system Sim_Multi/True dynamic system representation of a multirotor UAV/Force//Moment computation/Forces and moments generated by spinning propellers/Total airspeed (Body axes)/Inertial to Body ==
  DCM_ib : Inport
  Wind_i : Inport  Port=2
  Product : Product  Multiplication=Matrix(*)
  Reshape : Reshape  OutputDimensionality=Column vector (2-D)
  Reshape1 : Reshape  OutputDimensionality=Column vector (2-D)
  Wind_b : Outport
  wires:
  Reshape/1 -> Product/2
  Product/1 -> Reshape1/1
  Reshape1/1 -> Wind_b/1
  Wind_i/1 -> Reshape/1
  DCM_ib/1 -> Product/1  "DCM_ib"

== system Sim_Multi/Controller/Controller Structure/Inner-loop control only/PI Rate controller/Cross Product/Subsystem ==
  u : Inport
  v : Inport  Port=2
  Demux : Demux  Outputs=3
  Demux1 : Demux  Outputs=3
  Mux : Mux  Inputs=3
  Product : Product
  Product1 : Product
  Product2 : Product
  Positive elements : Outport
  wires:
  Mux/1 -> Positive elements/1
  v/1 -> Demux1/1
  u/1 -> Demux/1
  Demux/2 -> Product/1
  Demux1/3 -> Product/2
  Demux/3 -> Product1/1
  Demux1/1 -> Product1/2
  Demux/1 -> Product2/1
  Demux1/2 -> Product2/2
  Product/1 -> Mux/1
  Product1/1 -> Mux/2
  Product2/1 -> Mux/3

== system Sim_Multi/Controller/Controller Structure/Inner-loop control only/PI Rate controller/Cross Product/Subsystem1 ==
  u : Inport
  v : Inport  Port=2
  Demux : Demux  Outputs=3
  Demux1 : Demux  Outputs=3
  Mux : Mux  Inputs=3
  Product : Product
  Product1 : Product
  Product2 : Product
  Negative elements : Outport
  wires:
  Mux/1 -> Negative elements/1
  v/1 -> Demux1/1
  u/1 -> Demux/1
  Product/1 -> Mux/1
  Product1/1 -> Mux/2
  Product2/1 -> Mux/3
  Demux/3 -> Product/1
  Demux1/2 -> Product/2
  Demux/1 -> Product1/1
  Demux1/3 -> Product1/2
  Demux/2 -> Product2/1
  Demux1/1 -> Product2/2

== system Sim_Multi/Controller/Controller Structure/Inner-loop control only/PI Rate controller/Gain Kff/Create diagonal 3x3 matrix ==
  Vector : Inport
  Constant2 : Constant  Value=0
  Demux : Demux  Outputs=3
  Subsystem9 : Subsystem
  Matrix : Outport
  wires:
  Demux/1 -> Subsystem9/1(C_11)
  Demux/2 -> Subsystem9/5(C_22)
  Vector/1 -> Demux/1
  Constant2/1 -> Subsystem9/8(C_32), Subsystem9/7(C_31), Subsystem9/6(C_23), Subsystem9/4(C_21), Subsystem9/3(C_13), Subsystem9/2(C_12)
  Subsystem9/1(Diag) -> Matrix/1
  Demux/3 -> Subsystem9/9(C_33)

== system Sim_Multi/Controller/Controller Structure/Inner-loop control only/PI Rate controller/Gain Ki/Create diagonal 3x3 matrix ==
  Vector : Inport
  Constant2 : Constant  Value=0
  Demux : Demux  Outputs=3
  Subsystem9 : Subsystem
  Matrix : Outport
  wires:
  Demux/1 -> Subsystem9/1(C_11)
  Demux/2 -> Subsystem9/5(C_22)
  Vector/1 -> Demux/1
  Constant2/1 -> Subsystem9/8(C_32), Subsystem9/7(C_31), Subsystem9/6(C_23), Subsystem9/4(C_21), Subsystem9/3(C_13), Subsystem9/2(C_12)
  Subsystem9/1(Diag) -> Matrix/1
  Demux/3 -> Subsystem9/9(C_33)

== system Sim_Multi/Controller/Controller Structure/Inner-loop control only/PI Rate controller/Gain Kp/Create diagonal 3x3 matrix ==
  Vector : Inport
  Constant2 : Constant  Value=0
  Demux : Demux  Outputs=3
  Subsystem9 : Subsystem
  Matrix : Outport
  wires:
  Demux/1 -> Subsystem9/1(C_11)
  Demux/2 -> Subsystem9/5(C_22)
  Vector/1 -> Demux/1
  Constant2/1 -> Subsystem9/8(C_32), Subsystem9/7(C_31), Subsystem9/6(C_23), Subsystem9/4(C_21), Subsystem9/3(C_13), Subsystem9/2(C_12)
  Subsystem9/1(Diag) -> Matrix/1
  Demux/3 -> Subsystem9/9(C_33)

== system Sim_Multi/True dynamic system representation of a multirotor UAV/6DOF model/Quat Strapdown Eq./Normalize/norm/dot_product ==
  u : Inport
  v : Inport  Port=2
  Product : Product  Multiplication=Matrix(*)  RndMeth=Zero
  Reshape : Reshape  OutputDimensionality=Column vector (2-D)
  Reshape1 : Reshape  OutputDimensionality=Column vector (2-D)
  transpose : Math  Operator=transpose  SaturateOnIntegerOverflow=on
  u.v : Outport
  wires:
  v/1 -> Reshape1/1
  u/1 -> Reshape/1
  Reshape/1 -> transpose/1
  transpose/1 -> Product/1
  Reshape1/1 -> Product/2
  Product/1 -> u.v/1

== system Sim_Multi/True dynamic system representation of a multirotor UAV/Force//Moment computation/Compute aerodynamic drag of the airframe in Body axes/Aerodynamic drag force/Nonzero airspeed/Normalize ==
  Input : Inport
  Divide : Product  Inputs=*/
  norm : Subsystem
  Output : Outport
  wires:
  Input/1 -> Divide/1, norm/1(u)
  norm/1(||u||) -> Divide/2
  Divide/1 -> Output/1

== system Sim_Multi/True dynamic system representation of a multirotor UAV/Force//Moment computation/Compute aerodynamic drag of the airframe in Body axes/Aerodynamic drag force/Nonzero airspeed/Surface area computation ==
  Airspeed (Body) : Inport
  Surface_params : Inport  Port=2
  Scaling factor computation : Subsystem
  Surface area computation : Subsystem
  Area : Outport
  wires:
  Surface_params/1 -> Scaling factor computation/2(Surface_params)
  Airspeed (Body)/1 -> Surface area computation/1(Airspeed (Body)), Scaling factor computation/1(Airspeed (Body))
  Scaling factor computation/1(Scaling factor) -> Surface area computation/2(Scaling factor)
  Surface area computation/1(Surface area) -> Area/1

== system Sim_Multi/True dynamic system representation of a multirotor UAV/Force//Moment computation/Compute aerodynamic drag of the airframe in Body axes/Aerodynamic drag force/Nonzero airspeed/u^2 ==
  u : Inport
  dot_product : Subsystem
  u^2 : Outport
  wires:
  u/1 -> dot_product/1(u), dot_product/2(v)
  dot_product/1(u.v) -> u^2/1

== system Sim_Multi/True dynamic system representation of a multirotor UAV/Force//Moment computation/Compute aerodynamic drag of the airframe in Body axes/Aerodynamic drag force/norm/dot_product ==
  u : Inport
  v : Inport  Port=2
  Product : Product  Multiplication=Matrix(*)  RndMeth=Zero
  Reshape : Reshape  OutputDimensionality=Column vector (2-D)
  Reshape1 : Reshape  OutputDimensionality=Column vector (2-D)
  transpose : Math  Operator=transpose  SaturateOnIntegerOverflow=on
  u.v : Outport
  wires:
  v/1 -> Reshape1/1
  u/1 -> Reshape/1
  Reshape/1 -> transpose/1
  transpose/1 -> Product/1
  Reshape1/1 -> Product/2
  Product/1 -> u.v/1

== system Sim_Multi/True dynamic system representation of a multirotor UAV/Force//Moment computation/Forces and moments generated by spinning propellers/For Each Subsystem/Actuator dynamics/Continuous Integrator with dynamic upper//lower limits ==
  Integrator input : Inport
  Lower limit : Inport  Port=2
  Upper limit : Inport  Port=3
  Compare To Zero : simulink/Logic and Bit Operations/Compare To Zero  relop=<  OutDataTypeStr=uint8  ZeroCross=off
  Compare To Zero1 : simulink/Logic and Bit Operations/Compare To Zero  relop=>  OutDataTypeStr=uint8  ZeroCross=off
  Constant : Constant  Value=0
  Integrator : Integrator  InitialCondition=rpm_init
  Logical Operator : Logic  Operator=OR  AllPortsSameDT=off  OutDataTypeStr=boolean
  Logical Operator1 : Logic  Operator=OR  AllPortsSameDT=off  OutDataTypeStr=boolean
  Logical Operator2 : Logic  AllPortsSameDT=off  OutDataTypeStr=boolean
  Relational Operator : RelationalOperator  Operator=<=  OutDataTypeStr=boolean  RndMeth=Nearest
  Relational Operator1 : RelationalOperator  OutDataTypeStr=boolean  RndMeth=Nearest
  Saturation Dynamic : simulink/Discontinuities/Saturation Dynamic  OutMin=[]  OutMax=[]  OutDataTypeStr=Inherit: Same as second input  OutDataType=fixdt(1, 16)  OutScaling=2^-10  DoSatur=off
  Switch : Switch  Criteria=u2 > Threshold
  Output : Outport
  wires:
  Integrator input/1 -> Switch/1, Compare To Zero1/1, Compare To Zero/1
  Constant/1 -> Switch/3
  Switch/1 -> Integrator/1
  Relational Operator/1 -> Logical Operator/1
  Compare To Zero/1 -> Logical Operator/2
  Upper limit/1 -> Relational Operator/2, Saturation Dynamic/1
  Lower limit/1 -> Saturation Dynamic/3, Relational Operator1/2
  Compare To Zero1/1 -> Logical Operator1/1
  Relational Operator1/1 -> Logical Operator1/2
  Logical Operator1/1 -> Logical Operator2/2
  Logical Operator/1 -> Logical Operator2/1
  Logical Operator2/1 -> Switch/2
  Saturation Dynamic/1 -> Output/1
  Integrator/1 -> Relational Operator/1, Saturation Dynamic/2, Relational Operator1/1

== system Sim_Multi/True dynamic system representation of a multirotor UAV/Force//Moment computation/Forces and moments generated by spinning propellers/For Each Subsystem/Cross Product/Subsystem ==
  omega : Inport
  r : Inport  Port=2
  Demux : Demux  Outputs=3
  Demux1 : Demux  Outputs=3
  Mux : Mux  Inputs=3
  Product : Product
  Product1 : Product
  Product2 : Product
  Positive elements : Outport
  wires:
  Mux/1 -> Positive elements/1
  r/1 -> Demux1/1
  omega/1 -> Demux/1
  Demux/2 -> Product/1
  Demux1/3 -> Product/2
  Demux/3 -> Product1/1
  Demux1/1 -> Product1/2
  Demux/1 -> Product2/1
  Demux1/2 -> Product2/2
  Product/1 -> Mux/1  "u2*v3"
  Product1/1 -> Mux/2  "u3*v1"
  Product2/1 -> Mux/3  "u1*v2"

== system Sim_Multi/True dynamic system representation of a multirotor UAV/Force//Moment computation/Forces and moments generated by spinning propellers/For Each Subsystem/Cross Product/Subsystem1 ==
  omega : Inport
  r : Inport  Port=2
  Demux : Demux  Outputs=3
  Demux1 : Demux  Outputs=3
  Mux : Mux  Inputs=3
  Product : Product
  Product1 : Product
  Product2 : Product
  Negative elements : Outport
  wires:
  Mux/1 -> Negative elements/1
  r/1 -> Demux1/1
  omega/1 -> Demux/1
  Product/1 -> Mux/1  "u3*v2"
  Product1/1 -> Mux/2  "u1*v3"
  Product2/1 -> Mux/3  "u2*v1"
  Demux/3 -> Product/1
  Demux1/2 -> Product/2
  Demux/1 -> Product1/1
  Demux1/3 -> Product1/2
  Demux/2 -> Product2/1
  Demux1/1 -> Product2/2
